simulink model "template_kernel"  (R2019b)
settings: Solver=VariableStepAuto  StartTime=0.0  StopTime=10.0  RelTol=1e-3
undefined symbols (not defined in the file): xc7vx485tffg1157
libraries: ModelComposer x2, simulink x1
settings Model: Creator=viswanad  LastModifiedBy=abehbood

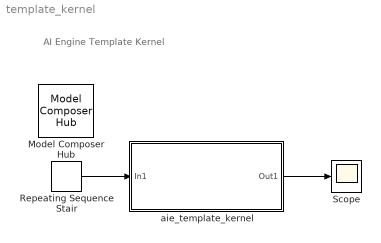
== system template_kernel ==
  note: AI Engine Template Kernel
  Model Composer Hub : ModelComposer/Model Composer Hub  CodeGeneration=off  SubsystemName=aie_template_kernel  TargetDirectory=./code_1  ExportType=AI Engines  IpVendor=xilinx.com  IpLibrary=hls  IpVersion=1.0  IpHWLanguage=Verilog  AieCompilerOptions={}  CreateTestbench=on  TestbenchStackSize=10  RunAieSim=on  AieSimTimeout=50000  LaunchVitisAnalyzer=off  RunX86Sim=off  X86SimTimeout=10  ProjDevice=xc7vx485tffg1157-1  ProjDevicePart=xc7vx485tffg1157-1  SamplePeriod=-1  ClockFrequency=200  DataPathParallelism=1
  Repeating Sequence Stair : simulink/Sources/Repeating Sequence Stair  OutValues=[1:20].'  tsamp=1  OutMin=[]  OutMax=[]  OutDataTypeStr=int32  OutputDataTypeScalingMode=int32  OutDataType=fixdt(0,8)  ConRadixGroup=Best Precision: Vector-wise  OutScaling=2^-12
  Scope : Scope
  aie_template_kernel : Subsystem
  wires:
  Repeating Sequence Stair/1 -> aie_template_kernel/1(In1)
  aie_template_kernel/1(Out1) -> Scope/1

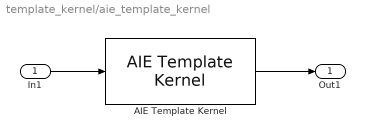
== system template_kernel/aie_template_kernel ==
  In1 : Inport
  AIE Template Kernel : ModelComposer/AIE Template Kernel  KernelAllAttrs=|  PortNames={'i1'; 'o1'}  PortSerializedTypes={'{P{Tinput_stream{1{t{ET}}}}}'; '{P{Toutput_stream{1{t{ET}}}}}'}  PortWindowSizes={0.000000000000000000e+00; 0.000000000000000000e+00}  PortWindowMargins={0.000000000000000000e+00; 0.000000000000000000e+00}  PortSynchronicities={'auto'; 'auto'}  PortSignalSizes={0.000000000000000000e+00; 1.000000000000000000e+00}  FunctionTemplateSpecKind=implicit  FunctionTemplateParamNames={'T'; 'N'}  FunctionTemplateParamKinds={'type'; 'nontype'}  FunctionTemplateParamTypes={'typename'; 'int'}  FunctionTemplateParamValues={'int32', '12'}  FunctionIndex=1  FunctionTabVisible=on  FunctionTemplateParamsVisible=on  FunctionDeclTypeOptions=|  FunctionDecl=|  FunctionTemplateParams={ 'T', 'typename', 'int32'; 'N', 'int', '12' }  FunctionTemplateParamsEnables={'off', 'off', 'on';'off', 'off', 'on'}  PortAttrs={ 'input', 'i1', 'input_stream< T > *', '', '', '', ''; 'output', 'o1', 'output_stream< T > *', '', '', '', '1' }  PortAttrsEnables={'off', 'off', 'off', 'off', 'off', 'off', 'off';'off', 'off', 'off', 'off', 'off', 'off', 'on'}  KernelHeaderFile=src/template_kernel.h  KernelFunction=template_func  KernelSourceFile=src/template_kernel.cpp  KernelSearchPaths={}  PreProcOptions={}  CoreRuntimeRatio=0.9
      KernelAllAttrs=|
      | s[12;12;9;9;19;14;21;23;24;21;12;24;26;26;26;27;28;9;21;23;23;23;24;25;14;19;19;29]@FunctionNameDeclFileNamePortNamesPortTypesPortSerializedTypesPortDirectionsPortWindowSizeEnablesPortWindowMarginEnablesPortSynchronicityEnablesPortSignalSizeEnablesFunctionDeclFunctionTemplateSpecKindFunctionTemplateParamNamesFunctionTemplateParamKindsFunctionTemplateParamTypesFunctionTemplateParamValuesFunctionTemplateParamEnablesClassDeclClassTemplateSpecKindClassTemplateParamNamesClassTemplateParamKindsClassTemplateParamTypesClassTemplateParamValuesClassTemplateParamEnablesClassCtorDeclsClassCtorParamNamesClassCtorParamTypesClassCtorParamSerializedTypes[1 1]@C[28 1]@t13@template_funct27@../../src/template_kernel.hC[2 1]@t2@i1t2@o1C[2 1]@t19@input_stream< T > *t20@output_stream< T > *C[2 1]@t28@{P{Tinput_stream{1{t{ET}}}}}t29@{P{Toutput_stream{1{t{ET}}}}}C[2 1]@t5@inputt6@outputC[2 1]@l0@l0@C[2 1]@l0@l0@C[2 1]@l0@l0@C[2 1]@l0@l1@t99@template < typename T, int N > 
      | void template_func(input_stream< T > * i1, output_stream< T > * o1)t8@implicitC[2 1]@t1@Tt1@NC[2 1]@t4@typet7@nontypeC[2 1]@t8@typenamet3@intC[2 1]@nnC[2 1]@l1@l1@nne[0 1]@e[0 1]@e[0 1]@e[0 1]@e[0 1]@e[0 1]@e[0 1]@e[0 1]@e[0 1]@
      FunctionDeclTypeOptions=|
      | C[1 1]@t99@template < typename T, int N > 
      | void template_func(input_stream< T > * i1, output_stream< T > * o1)
      FunctionDecl=|
      | template < typename T, int N > 
      | void template_func(input_stream< T > * i1, output_stream< T > * o1)
  Out1 : Outport
  wires:
  In1/1 -> AIE Template Kernel/1
  AIE Template Kernel/1 -> Out1/1
